simulink model "Lab06_tostudents_useMe_2023b"  (R2023b)
settings: Solver=FixedStepAuto  StartTime=0.0  StopTime=inf  RelTol=1e-3  EnableMultiTasking=on
InitFcn:
  | Ts = 0.01;
  | IniT = 8;
  | FilterGain = 0.02;
libraries: arduinolib x2
settings Model: ExtModeTrigDuration=2  Creator=bnewman  LastModifiedBy=Samantha Burton
settings SolverCC: AlgebraicLoopSolver=TrustRegion
settings DataIOCC: ReturnWorkspaceOutputs=off
settings OptimizationCC: PassReuseOutputArgsThreshold=0  MaxStackSize=64
settings DebuggingCC: ParameterTunabilityLossMsg=error  UnconnectedInputMsg=warning  UnconnectedOutputMsg=warning  UnconnectedLineMsg=warning  PregeneratedLibrarySubsystemCodeDiagnostic=none  ArithmeticOperatorsInVariantConditions=warning
settings HardwareCC: ProdBitPerInt=16  ProdBitPerPointer=16  ProdBitPerSizeT=16  ProdBitPerPtrDiffT=16  ProdLargestAtomicFloat=None  ProdWordSize=8  ProdLongLongMode=on  ProdHWDeviceType=Atmel->AVR
settings ModelReferenceCC: EnableRefExpFcnMdlSchedulingChecks=on
settings SFSimCC: SimUseLocalCustomCode=off  MATLABDynamicMemAlloc=off  CustomCodeUndefinedFunction=UseInterfaceOnly
settings RTWCC: Description=Embedded Coder  SystemTargetFile=ert.tlc  HardwareBoard=Arduino Uno  TemplateMakefile=ert_default_tmf  RTWVerbose=off  RTWUseLocalCustomCode=off  Toolchain=Arduino AVR  BuildConfiguration=Faster Runs  DLArmComputeVersion=19.05
settings CodeAppCC: ForceParamTrailComments=on  OperatorAnnotations=on  MangleLength=10
settings ERTTargetCC: ERTCustomFileBanners=off  SupportContinuousTime=on  SupportNonInlinedSFcns=on  RemoveResetFunc=off  SupportVariableSizeSignals=on  ModelStepFunctionPrototypeControlCompliant=off  ExtMode=on  ExtModeStaticAllocSize=250  ExtModeMexArgs='172.20.10.10' 0 17725  ERTSrcFileBannerTemplate=codertarget_code_template.cgt  ERTHdrFileBannerTemplate=codertarget_code_template.cgt  ERTDataSrcFileTemplate=codertarget_code_template.cgt  ERTDataHdrFileTemplate=codertarget_code_template.cgt
settings SettingsController: UseSoCProfilerForTargets=0

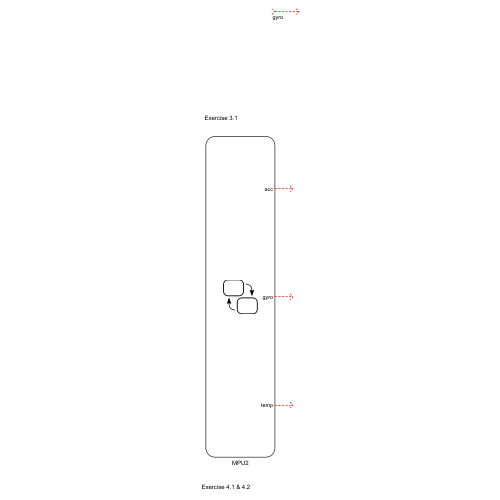
[thumbnail: Simulink's stored preview of the top-level diagram]
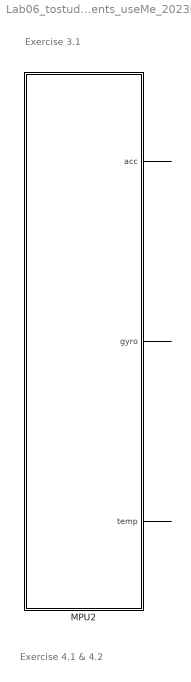
== system Lab06_tostudents_useMe_2023b ==
  note: Exercise 3.1
  note: Exercise 4.1 & 4.2
  MPU2 : Stateflow chart  TreatAsAtomicUnit=on
  wires:
  ? -> ?  "gyro"
  MPU2/1(acc) -> ?
  MPU2/2(gyro) -> ?
  MPU2/3(temp) -> ?

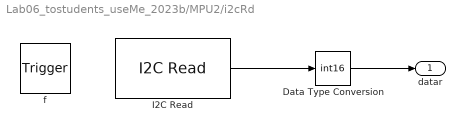
== system Lab06_tostudents_useMe_2023b/MPU2/i2cRd ==
  f : TriggerPort  TriggerType=function-call  VariantControl=Variant  SampleTime=inf
      settings: CopyFcn=Stateflow.SLINSF.SimulinkMan.removeBlockPreDeleteFcn  PreDeleteFcn=Stateflow.SLINSF.SimulinkMan.unsafePredeleteFcn
  Data Type Conversion : DataTypeConversion  OutDataTypeStr=int16  SaturateOnIntegerOverflow=off  RndMeth=Floor
  I2C Read : arduinolib/I2C Read  I2CModule=0  Mode=Master  SlaveAddress=hex2dec( '68' )  SlaveByteOrder=BigEndian  Direction=Receiver  RegisterAddressMode=on  RegisterAddress=hex2dec( '3b' )  SlaveDataType=uint16  DataLength=7  NoAck=off  RepeatedStart=off  OutputStatus=off  blockPlatform=arduino  SampleTime=-1
      settings: SourceProductName=Common
  datar : Outport  OutDataTypeStr=int16  Unit=1  PortDimensions=7  VectorParamsAs1DForOutWhenUnconnected=off
  wires:
  I2C Read/1 -> Data Type Conversion/1
  Data Type Conversion/1 -> datar/1

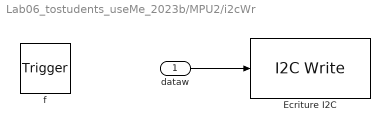
== system Lab06_tostudents_useMe_2023b/MPU2/i2cWr ==
  dataw : Inport  OutDataTypeStr=uint16  Unit=1  PortDimensions=1
  f : TriggerPort  TriggerType=function-call  VariantControl=Variant  SampleTime=-1
      settings: CopyFcn=Stateflow.SLINSF.SimulinkMan.removeBlockPreDeleteFcn  PreDeleteFcn=Stateflow.SLINSF.SimulinkMan.unsafePredeleteFcn
  Ecriture I2C : arduinolib/I2C Write  Priority=1  I2CModule=0  Mode=Master  SlaveAddress=hex2dec( '68' )  SlaveByteOrder=BigEndian  Direction=Transmitter  RegisterAddressMode=off  RegisterAddress=hex2dec( '6B' )  SlaveDataType=uint16  DataLength=1  NoAck=off  RepeatedStart=off  OutputStatus=off  blockPlatform=arduino
      settings: SourceProductName=Common
  wires:
  dataw/1 -> Ecriture I2C/1

== stateflow chart Lab06_tostudents_useMe_2023b/MPU2 ==
  state initialisation
    en:
    i2cWr(uint16(hex2dec( '6B00' )));%Power on
    i2cWr(uint16(hex2dec( '1B10' )));%gyro 0x10=1000°/s
    i2cWr(uint16(hex2dec( '1C08' )));%acce 0x08= 4G
    i2cWr(uint16(hex2dec( '1A06' )));%filtrage+actu 0x06= 19ms
    i2cWr(uint16(hex2dec( '3710' )));%INT_PIN_CFG
    i2cWr(uint16(hex2dec( '3800' )));%Interrupt Enable 0 désactivé
  state Lecture_acceleration3_axes
    during:
    val=i2cRd;
    acc=val(1:3);
    gyro=val(5:7);
    temp=val(4:4);
  state i2cWr(dataw) [function]
  state datar = i2cRd [function]
  (default) -> initialisation
  initialisation -> Lecture_acceleration3_axes
  data: dataw function_input uint16 size=1; datar function_output int16 size=7; acc output int16 size=3; gyro output int16 size=3; val local int16 size=7; temp output int16 size=1
